simulink model "prob1_214869"  (R2020a)
settings: Solver=VariableStepAuto  StartTime=0.0  StopTime=inf  RelTol=1e-3
settings Model: Creator=sonal  LastModifiedBy=sonal

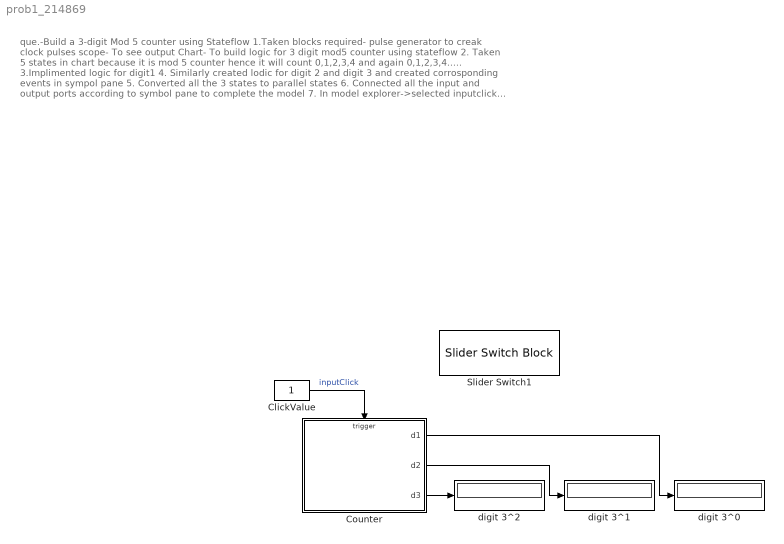
== system prob1_214869 ==
  note: que.-Build a 3-digit Mod 5 counter using Stateflow
      |
      | 1.Taken blocks required-
      | pulse generator to creak clock pulses
      | scope- To see output
      | Chart- To build logic for 3 digit mod5 counter using stateflow
      | 2. Taken 5 states in chart because it is mod 5 counter hence it will count
      | 0,1,2,3,4 and again 0,1,2,3,4.....
      | 3.Implimented logic for digit1
      | 4. Similarly created lodic for digit 2 and digit 3 and created corrosponding events in sympol pane
      | 5. Converted all the 3 states to parallel states
      | 6. Connected all the input and output ports according to symbol pane to complete the model
      | 7. In model explorer->selected inputclick in chart-> and trigger converted to rising edge
      | 8. Made stop time of simulation -inf
  ClickValue : Constant
  Counter : Stateflow chart  TreatAsAtomicUnit=on
  Slider Switch1 : SliderSwitchBlock  LabelPosition=Bottom
      settings: Values={{'Off', 'On'}, [0 1]}
  digit 3^0 : Display
  digit 3^1 : Display
  digit 3^2 : Display
  wires:
  Counter/3(d3) -> digit 3^2/1
  Counter/2(d2) -> digit 3^1/1
  ClickValue/1 -> Counter/Trigger  "inputClick"
  Counter/1(d1) -> digit 3^0/1

== stateflow chart prob1_214869/Counter ==
  settings: executeAtInitialization=1
  state digit1 [parallel]
    settings: executionOrder=1
    state one
      en: d1 = 1;
    state two
      en: d1 = 2;
    state zero
      en: d1 = 0;
    state three
      en: d1 = 3;
    state four
      en: d1 = 4;
    digit1.zero -> digit1.one : inputClick
    digit1.one -> digit1.two : inputClick
    (default) -> digit1.zero
    digit1.four -> digit1.zero : inputClick /{digit2.inc2;}
    digit1.two -> digit1.three : inputClick
    digit1.three -> digit1.four : inputClick
  state digit2 [parallel]
    settings: executionOrder=2
    state one
      en: d2 = 1;
    state two
      en: d2 = 2;
    state zero
      en: d2 = 0;
    state three
      en: d2 = 3;
    state four
      en: d2 = 4;
    digit2.zero -> digit2.one : inc2
    digit2.one -> digit2.two : inc2
    (default) -> digit2.zero
    digit2.four -> digit2.zero : inc2 /{digit3.inc3;}
    digit2.two -> digit2.three : inc2
    digit2.three -> digit2.four : inc2
  state digit3 [parallel]
    settings: executionOrder=3
    state one
      en: d3 = 1;
    state two
      en: d3 = 2;
    state zero
      en: d3 = 0;
    state four
      en: d3 = 4;
    state three
      en: d3 = 3;
    digit3.zero -> digit3.one : inc3
    digit3.one -> digit3.two : inc3
    (default) -> digit3.zero
    digit3.four -> digit3.zero : inc3
    digit3.two -> digit3.three : inc3
    digit3.three -> digit3.four : inc3
  data: d1 output size=1; d2 output size=1; d3 output size=1
  events: inc2 local EITHER_EDGE_EVENT; inc3 local EITHER_EDGE_EVENT; inputClick input RISING_EDGE_EVENT
